simulink model "MSDPwalkingrigid"  (R2019a)
settings: Solver=FixedStepAuto  StartTime=0.0  StopTime=500  FixedStep=Ts  RelTol=1e-3  EnableMultiTasking=on
undefined symbols (not defined in the file): f1_off, f2_off, f3_off, f4_off, f5_off, f6_off, Pull, trial, Ts, up, weight
libraries: speedgoatlib_IO183 x6, slrtlib x5, dspsigops x3, dspswit3 x1, dspstat3 x1, simulink x1
settings Model: Creator=vnalam  LastModifiedBy=vnalam
settings DataIOCC: LimitDataPoints=on  SaveFormat=StructureWithTime  ReturnWorkspaceOutputs=off
settings OptimizationCC: BlockReduction=off  OptimizeBlockIOStorage=off  BufferReuse=off  GlobalBufferReuse=off  ExpressionFolding=off  LocalBlockOutputs=off  LifeSpan=inf  OptimizeDataStoreBuffers=off  BusAssignmentInplaceUpdate=off
settings DebuggingCC: AllowSymbolicDim=off  SFUnexpectedBacktrackingDiag=warning  SFNoUnconditionalDefaultTransitionDiag=warning  SFExecutionAtInitializationDiag=none  ArithmeticOperatorsInVariantConditions=warning
settings HardwareCC: ProdBitPerPointer=32  ProdBitPerSizeT=32  ProdBitPerPtrDiffT=32  ProdLargestAtomicFloat=None  ProdWordSize=32  ProdLongLongMode=on  ProdHWDeviceType=Generic->32-bit x86 compatible
settings ModelReferenceCC: PropagateSignalLabelsOutOfModel=off
settings SFSimCC: SimUseLocalCustomCode=off
settings RTWCC: SystemTargetFile=slrt.tlc  TLCOptions=-axPCModelStackSizeKB=512  TemplateMakefile=slrt_default_tmf  Description=Simulink Real-Time  RTWUseLocalCustomCode=off  CodeExecutionProfiling=on  RTWCompilerOptimization=on
settings CodeAppCC: StateflowObjectComments=on
settings SimulinkRealTimeCC: PreserveStateflowLocalDataDimensions=off  xPCisDownloadable=off
settings ConfigComp: CovMetricSettings=dw  CovHtmlReporting=on  CovSaveCumulativeToWorkspaceVar=on  CovSaveSingleToWorkspaceVar=on  CovExternalEMLEnable=off

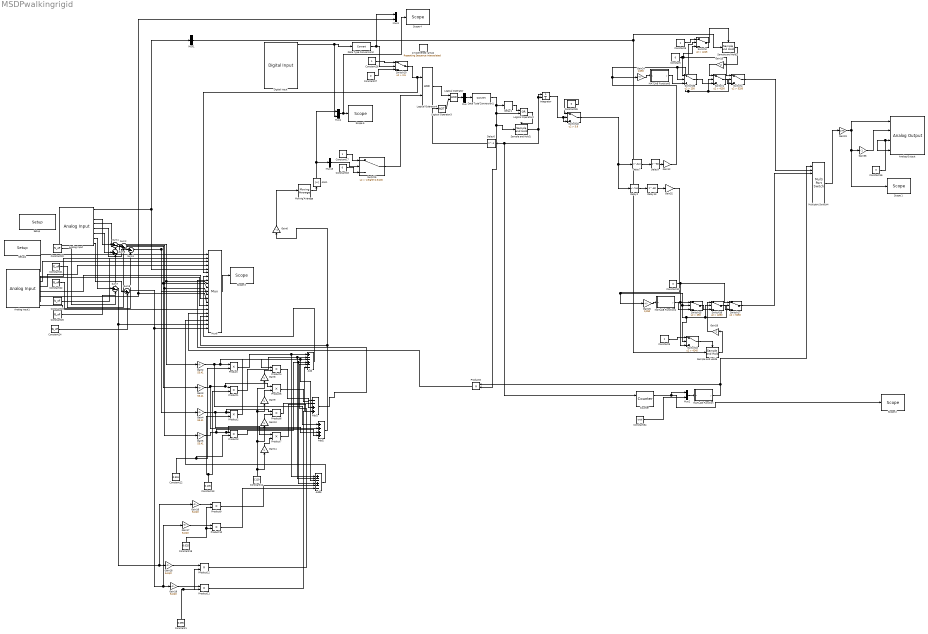
== system MSDPwalkingrigid ==
  Abs1 : Abs
  Add : Sum  Inputs=+--+--
  Add1 : Sum  Inputs=--++
  Add2 : Sum  Inputs=++++
  Add3 : Sum  Inputs=+--+--
  Analog Input : speedgoatlib_IO183/Analog Input  Priority=0  parModuleId=1  parSampTime=Ts  parPciSlot=-1  parAdChannelLow=1  parAdChannelHigh=8
      settings: SourceProductName=Simulink Real-Time: Speedgoat Library
  Analog Input1 : speedgoatlib_IO183/Analog Input  Priority=0  parModuleId=2  parSampTime=Ts  parPciSlot=-1  parAdChannelLow=1  parAdChannelHigh=8
      settings: SourceProductName=Simulink Real-Time: Speedgoat Library
  Analog Output : speedgoatlib_IO183/Analog Output  parModuleId=1  parSampTime=-1  parDaSimult=on  parPciSlot=-1  parDaChannels=[1 2 3 4]  parDaInit=[0 0 0 0]  parDaReset=[0 0 0 0]
      settings: SourceProductName=Simulink Real-Time: Speedgoat Library
  Constant{,10,16,18,27,35} (6 alike) : Constant  Value=0  SampleTime=Ts
  Constant1 : Constant  Value=0.095  SampleTime=-1
  Constant11 : Constant  Value=0.110  SampleTime=-1
  Constant12 : Constant  Value=0.315  SampleTime=-1
  Constant13 : Constant  Value=0.105  SampleTime=-1
  Constant{5..6,17,26} (4 alike) : Constant  SampleTime=Ts
  Constant19 : Constant  Value=0.025  SampleTime=-1
  Constant20 : Constant  Value=f1_off  SampleTime=Ts
  Constant21 : Constant  Value=f2_off  SampleTime=Ts
  Constant22 : Constant  Value=f3_off  SampleTime=Ts
  Constant23 : Constant  Value=f4_off  SampleTime=Ts
  Constant24 : Constant  Value=f6_off  SampleTime=Ts
  Constant25 : Constant  Value=f5_off  SampleTime=Ts
  Constant34 : Constant  Value=trial  SampleTime=Ts
  Counter : dspswit3/Counter  Direction=Up  CountEvent=Rising edge  CounterSize=User defined  MaxCount=255  InitialCount=0  Output=Count and Hit  HitValue=32  ResetInput=on  SamplesPerFrame=1  Ts=1  CntDtype=double  HitDtype=Boolean
  Data Type Conversion1 : DataTypeConversion
  Data Type Conversion2 : DataTypeConversion
  Delay1 : Delay  DelayLength=12000  InitialCondition=0  SampleTime=Ts
  Delay13 : Delay  DelayLength=60  InitialCondition=0  SampleTime=Ts
  Delay2 : Delay  DelayLength=780  InitialCondition=0  SampleTime=Ts
  Delay6 : Delay  DelayLength=1  InitialCondition=0  SampleTime=Ts
  Delay7 : Delay  DelayLength=840  InitialCondition=0  SampleTime=Ts
  Delay9 : Delay  DelayLength=60  InitialCondition=0  SampleTime=Ts
  Digital Input : speedgoatlib_IO183/Digital Input  parModuleId=2  parSampTime=-1  parPciSlot=-1  parDiChannels=[9 10 11 12 13 14 15 16]
      settings: SourceProductName=Simulink Real-Time: Speedgoat Library
  Gain{8..11} (4 alike) : Gain
  Gain12 : Gain  Gain=2000
  Gain15 : Gain  Gain=-2
  Gain{16..19} (4 alike) : Gain  Gain=54.8/2
  Gain{2..5} (4 alike) : Gain  Gain=53.41
  Gain23 : Gain  Gain=1/40
  Gain24 : Gain  Gain=1/250
  Gain25 : Gain  Gain=1/250
  Gain26 : Gain  Gain=-2
  Gain32 : Gain  Gain=2000
  Gain36 : Gain  Gain=-1
  Gain6 : Gain  Gain=-1
  Integrator : Integrator  ExternalReset=rising
  Logical Operator : Logic  AllPortsSameDT=off  OutDataTypeStr=boolean
  Logical Operator2 : Logic  Operator=OR  AllPortsSameDT=off  OutDataTypeStr=boolean
  Logical Operator3 : Logic  Operator=NOT  AllPortsSameDT=off  OutDataTypeStr=boolean
  Logical Operator4 : Logic  AllPortsSameDT=off  OutDataTypeStr=boolean
  MATLAB Function : MATLAB Function  TreatAsAtomicUnit=on
  MATLAB Function4 : MATLAB Function  TreatAsAtomicUnit=on
  MATLAB Function5 : MATLAB Function  TreatAsAtomicUnit=on
  Moving Average : dspstat3/Moving Average  Method=Sliding window  ForgettingFactorPort=off  SpecifyWindowLength=on  WindowLength=4  ForgettingFactor=0.9  SimulateUsing=Code generation
  Multiport Switch4 : MultiPortSwitch  Inputs=9
  Mux : Mux  Inputs=1
  Mux1 : Mux  Inputs=1
  Mux13 : Mux  Inputs=1
  Mux2 : Mux  Inputs=2
  Mux3 : Mux  Inputs=2
  Mux4 : Mux  Inputs=2
  Mux6 : Mux  Inputs=21
      settings: DisplayOption=signals
  Product{,1..12} (13 alike) : Product
  Sample and Hold1 : dspsigops/Sample and Hold  trig=Rising edge  initCond=0  latchinput=off
  Sample and Hold2 : dspsigops/Sample and Hold  trig=Rising edge  initCond=0  latchinput=off
  Sample and Hold5 : dspsigops/Sample and Hold  trig=Rising edge  initCond=0  latchinput=off
  Scope 1 : slrtlib/Displays and Logging/Scope   scopeno=2  scopetype=Target  autostart=on  viewmode=Graphical sliding  formatstr='%15.6f'  grid=on  ylimits=[0,0]  nosamples=10000  noprepostsamples=0  interleave=1  triggermode=FreeRun  triggersignal=1  trigsignalfromport=off  triggerlevel=0.0  triggerslope=Either  triggerscope=1  triggersample=0  filename=tot303.dat  mode=Lazy  writesize=512  autorestart=off  dynamicfilemode=off  maxwritefilesize=512*1024^2
  Scope 2 : slrtlib/Displays and Logging/Scope   scopeno=1  scopetype=Target  autostart=on  viewmode=Numerical  formatstr='%15.6f'  grid=on  ylimits=[0,0]  nosamples=100  noprepostsamples=0  interleave=1  triggermode=FreeRun  triggersignal=1  trigsignalfromport=off  triggerlevel=0.0  triggerslope=Either  triggerscope=1  triggersample=0  filename=tot303.dat  mode=Lazy  writesize=512  autorestart=off  dynamicfilemode=off  maxwritefilesize=512*1024^2
  Scope 3 : slrtlib/Displays and Logging/Scope   scopeno=3  scopetype=File  autostart=on  viewmode=Graphical redraw  formatstr='%15.6f'  grid=on  ylimits=[0,0]  nosamples=800000  noprepostsamples=0  interleave=1  triggermode=FreeRun  triggersignal=1  trigsignalfromport=off  triggerlevel=0.0  triggerslope=Either  triggerscope=1  triggersample=0  filename=vwdud.dat  mode=Commit  writesize=1024  autorestart=off  dynamicfilemode=off  maxwritefilesize=512*1024^2
  Scope 4 : slrtlib/Displays and Logging/Scope   scopeno=4  scopetype=Target  autostart=on  viewmode=Graphical sliding  formatstr='%15.6f'  grid=on  ylimits=[0,0]  nosamples=20000  noprepostsamples=0  interleave=1  triggermode=FreeRun  triggersignal=1  trigsignalfromport=off  triggerlevel=0.0  triggerslope=Either  triggerscope=1  triggersample=0  filename=tot303.dat  mode=Lazy  writesize=512  autorestart=off  dynamicfilemode=off  maxwritefilesize=512*1024^2
  Scope 5 : slrtlib/Displays and Logging/Scope   scopeno=5  scopetype=Target  autostart=on  viewmode=Numerical  formatstr='%15.6f'  grid=on  ylimits=[0,0]  nosamples=100  noprepostsamples=0  interleave=1  triggermode=FreeRun  triggersignal=1  trigsignalfromport=off  triggerlevel=0.0  triggerslope=Either  triggerscope=1  triggersample=0  filename=tot303.dat  mode=Lazy  writesize=512  autorestart=off  dynamicfilemode=off  maxwritefilesize=512*1024^2
  Setup : speedgoatlib_IO183/Setup  parModuleId=1  parPciSlot=-1  parDaSimult=on  parAdCoupling=Single Ended  parAdRange=+-10V  parAdChannelLow=1  parAdChannelHigh=8  parDaChannels=[1:4]  parDaRange=0..5V  parDaInit=[0]  parDaReset=[0]  parDoChannels=[1:8]  parDoInit=[0]  parDoReset=[1]  parDiChannels=[9:16]  parIOPullReferenceFront=Pull-up (3.3V)  parIOPullReferenceRear=Pull-up (3.3V)
      settings: SourceProductName=Simulink Real-Time: Speedgoat Library
  Setup1 : speedgoatlib_IO183/Setup  parModuleId=2  parPciSlot=-1  parDaSimult=on  parAdCoupling=Single Ended  parAdRange=+-10V  parAdChannelLow=1  parAdChannelHigh=8  parDaChannels=[1:4]  parDaRange=0..5V  parDaInit=[0]  parDaReset=[0]  parDoChannels=[1:8]  parDoInit=[0]  parDoReset=[1]  parDiChannels=[9:16]  parIOPullReferenceFront=Pull-up (3.3V)  parIOPullReferenceRear=Pull-up (3.3V)
      settings: SourceProductName=Simulink Real-Time: Speedgoat Library
  Sum{1..3,6..8} (6 alike) : Sum  Inputs=|+-
  Switch1 : Switch  Criteria=u2 > Threshold  Threshold=4250
  Switch10 : Switch  Criteria=u2 > Threshold  Threshold=0.5
  Switch15 : Switch  Criteria=u2 > Threshold  Threshold=250
  Switch16 : Switch  Criteria=u2 > Threshold  Threshold=4250
  Switch17 : Switch  Criteria=u2 > Threshold  Threshold=5250
  Switch18 : Switch  Criteria=u2 > Threshold  Threshold=4245
  Switch2 : Switch  Criteria=u2 > Threshold  Threshold=4245
  Switch36 : Switch  Criteria=u2 > Threshold  Threshold=250
  Switch4 : Switch  Criteria=u2 > Threshold  Threshold=5250
  Switch40 : Switch  Criteria=u2 > Threshold  Threshold=5.9
  Switch5 : Switch  Criteria=u2 > Threshold  Threshold=weight*2.5/100
  smoothened ramp2 : simulink/Sources/Repeating Sequence Interpolated  OutValues="[0 1 1 0  0 ].'"  TimeValues=[0 0.0001 1.001 1.002 6.5].'  LookUpMeth=Interpolation-Use End Values  tsamp=Ts  OutMin=[]  OutMax=[]  OutDataTypeStr=double  OutputDataTypeScalingMode=double  OutDataType=fixdt(0,8)  OutScaling=2^-10
  wires:
  Mux6/1 -> Scope 3/1
  Gain2/1 -> Add2/1, Product4/1, Product/1
  Gain3/1 -> Add2/2, Product5/1, Product1/1
  Gain4/1 -> Add2/3, Product6/1, Product2/1
  Gain5/1 -> Add2/4, Product7/1, Product3/1
  Constant11/1 -> Gain8/1, Gain9/1, Gain10/1, Gain11/1
  Gain8/1 -> Product4/2
  Gain9/1 -> Product5/2
  Gain10/1 -> Product6/2
  Gain11/1 -> Product7/2
  Product/1 -> Add3/1, Add/1
  Product1/1 -> Add3/2, Add/2
  Product2/1 -> Add3/3, Add/3
  Product3/1 -> Add/4, Add3/4
  Product4/1 -> Add1/1
  Product6/1 -> Add1/3
  Product5/1 -> Add1/2
  Product7/1 -> Add1/4
  Constant13/1 -> Product2/2, Product1/2
  Constant12/1 -> Product3/2, Product/2
  Add/1 -> Mux6/7
  Add1/1 -> Mux6/8
  Constant17/1 -> Switch5/1
  Constant18/1 -> Switch5/3
  Mux13/1 -> Switch5/2
  Data Type Conversion2/1 -> Mux3/1, Switch10/2
  Constant26/1 -> Switch10/1
  Sum1/1 -> Gain2/1, Mux6/9
  Sum2/1 -> Gain3/1, Mux6/10
  Sum3/1 -> Mux6/11, Gain4/1
  Sum6/1 -> Gain5/1, Mux6/12
  Gain16/1 -> Product9/1
  Constant1/1 -> Product12/2, Product11/2
  Gain17/1 -> Product10/1
  Gain18/1 -> Product12/1
  Gain19/1 -> Product11/1
  Product12/1 -> Add/5
  Product11/1 -> Add/6
  Sum8/1 -> Mux6/21, Gain17/1, Gain19/1
  Analog Input1/2 -> Mux6/2
  Analog Input1/3 -> Mux6/3
  Analog Input1/7 -> Mux6/15
  Analog Input1/8 -> Mux6/16
  Analog Input1/1 -> Mux6/1
  Abs1/1 -> Mux4/1, Mux13/1
  Gain6/1 -> Moving Average/1
  Switch5/1 -> Logical Operator4/2
  Mux/1 -> Data Type Conversion1/1
  Delay1/1 -> Logical Operator2/1
  Logical Operator2/1 -> Sample and Hold1/Trigger
  Sample and Hold1/1 -> Counter/1, Delay6/1, Integrator/1, Integrator/2
  Logical Operator/1 -> Mux/1
  Logical Operator3/1 -> Logical Operator/2
  Delay6/1 -> Logical Operator3/1
  Gain12/1 -> Switch36/2, Switch4/2, Switch1/2, Switch2/2, Gain24/1
  Data Type Conversion1/1 -> Product8/2, Sample and Hold1/1, Logical Operator2/2, Delay1/1
  Switch1/1 -> Switch4/3
  Counter/1 -> Mux2/1, Scope 2/1
  MATLAB Function/1(y) -> Multiport Switch4/1, Product8/1
  Product8/1 -> Mux6/17
  Gain23/1 -> Scope 1/1, Gain36/1, Analog Output/1
  Analog Input1/5 -> Mux6/13
  Constant/1 -> Switch36/1, Switch2/3, Switch4/1
  Constant6/1 -> Switch2/1
  Switch2/1 -> Sample and Hold2/Trigger
  Sample and Hold2/1 -> Gain15/1
  Gain15/1 -> Switch1/1
  Add2/1 -> Gain6/1, Mux6/18
  Constant16/1 -> Analog Output/4, Analog Output/3
  Gain25/1 -> MATLAB Function4/1(u)
  Constant10/1 -> Switch17/1, Switch18/3, Switch15/1
  Switch16/1 -> Switch17/3
  Switch15/1 -> Switch16/3
  Switch18/1 -> Sample and Hold5/Trigger
  Constant5/1 -> Switch18/1
  Sample and Hold5/1 -> Gain26/1
  Gain26/1 -> Switch16/1
  MATLAB Function4/1(y) -> Switch15/3
  Mux1/1 -> Sample and Hold5/1, Sample and Hold2/1
  Analog Input1/4 -> Mux6/4
  Constant27/1 -> Switch10/3
  Switch10/1 -> Mux6/6, Logical Operator4/1
  Constant19/1 -> Product9/2, Product10/2
  Product9/1 -> Add3/5
  Product10/1 -> Add3/6
  Add3/1 -> Mux6/19
  Analog Input/3 -> Sum1/1
  Analog Input/4 -> Sum2/1
  Analog Input/5 -> Sum3/1
  Analog Input/6 -> Sum6/1
  Constant20/1 -> Sum1/2
  Constant21/1 -> Sum2/2
  Constant22/1 -> Sum3/2
  Constant23/1 -> Sum6/2
  Analog Input/7 -> Sum7/1
  Constant25/1 -> Sum7/2
  Analog Input/8 -> Sum8/1
  Constant24/1 -> Sum8/2
  Logical Operator4/1 -> Logical Operator/1
  Switch4/1 -> Multiport Switch4/2
  Switch17/1 -> Multiport Switch4/3
  Multiport Switch4/1 -> Gain23/1
  Delay7/1 -> Delay9/1
  Switch40/1 -> Delay2/1, Delay7/1
  Gain32/1 -> Gain25/1, Switch18/2, Switch17/2, Switch16/2, Switch15/2
  Delay13/1 -> Gain32/1
  Analog Input/1 -> Mux6/5, Mux1/1
  Mux2/1 -> MATLAB Function/1(u)
  Constant34/1 -> Mux2/2
  Delay9/1 -> Gain12/1
  Gain24/1 -> MATLAB Function5/1(u)
  MATLAB Function5/1(y) -> Switch36/3
  Switch36/1 -> Switch1/3
  Integrator/1 -> Switch40/3, Switch40/2
  Constant35/1 -> Switch40/1
  Sum7/1 -> Mux6/20, Gain16/1, Gain18/1
  Gain36/1 -> Analog Output/2
  Analog Input1/6 -> Mux3/2, Mux6/14
  Mux4/1 -> Scope 4/1, Scope 5/1
  Digital Input/1 -> Mux4/2, Data Type Conversion2/1
  Moving Average/1 -> Abs1/1
  Delay2/1 -> Delay13/1

== matlab function MSDPwalkingrigid/MATLAB Function5 ==
  data: u input; y output
function y = fcn(u)
%#codegen
y=3*((30*u^2-60*u^3+30*u^4))*2000/250;

== matlab function MSDPwalkingrigid/MATLAB Function4 ==
  data: u input; y output
function y = fcn(u)
%#codegen
y=0*((30*u^2-60*u^3+30*u^4))*2000/250;

== matlab function MSDPwalkingrigid/MATLAB Function ==
  data: u input; y output
function y = fcn(u)
%#codegen
y=0;


if u(1)==1
    y=2;
elseif u(1)==2
    y=1;
elseif u(1)==3
    y=1;
elseif u(1)==4
    y=2;
elseif u(1)==5
    y=1;
elseif u(1)==6
    y=2;
elseif u(1)==7
    y=1;
elseif u(1)==8
    y=2;
elseif u(1)==9
    y=1;
elseif u(1)==10
    y=2;
elseif u(1)==11
    y=1;
elseif u(1)==12
    y=1;
elseif u(1)==13
    y=2;
elseif u(1)==14
    y=2;
elseif u(1)==15
    y=1;
elseif u(1)==16
    y=2;
elseif u(1)==17
    y=1;
elseif u(1)==18
    y=2;
elseif u(1)==19
    y=1;
elseif u(1)==20
    y=2;    
end
end
